simulink model "power_1phPWM"  (Simulink 6.0)
settings: Solver=VariableStepDiscrete  SolverMode=SingleTasking  StartTime=0.0  StopTime=0.1  MaxStep=Ts  RelTol=1e-3
InitFcn:
  | Ts=1/60/3240;
libraries: powerlib x28, powerlib_extras x3
settings Model: Creator=patrice  LastModifiedBy=batserve  ExtModeTrigMode=oneshot  ExtModeArmWhenConnect=off  ExtModeAutoUpdateStatusClock=off
settings DataIOCC: LimitDataPoints=off  SignalLoggingName=sigsOut
settings OptimizationCC: BlockReduction=off  BooleanDataType=off
settings DebuggingCC: CheckExecutionContextPreStartOutputMsg=on  CheckExecutionContextRuntimeOutputMsg=on  SolverPrmCheckMsg=none
settings HardwareCC: TargetUnknown=on
settings RTWCC: TemplateMakefile=grt_unix.tmf

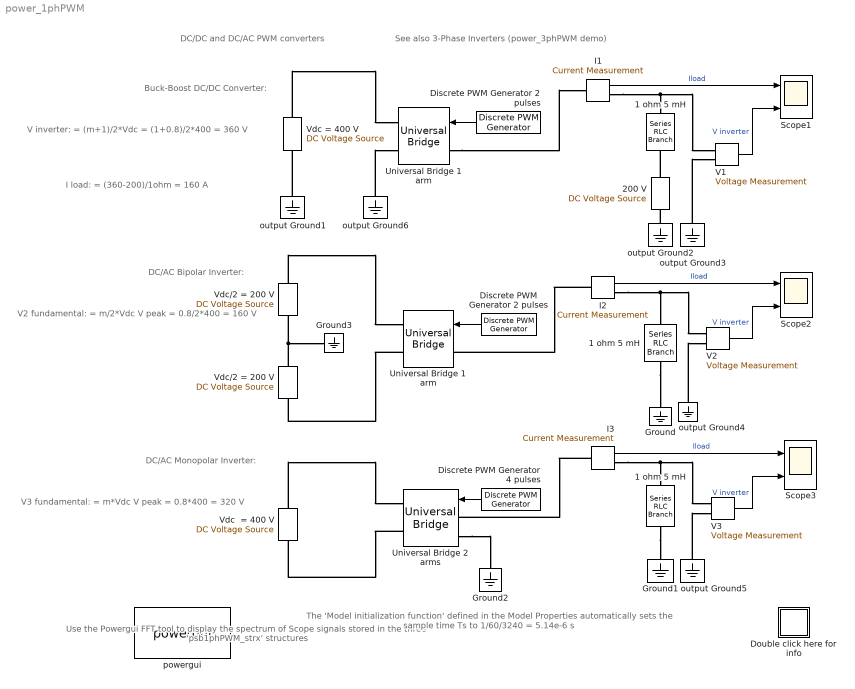
== system power_1phPWM ==
  note: V3 fundamental:
      |     = m*Vdc V peak
      |     = 0.8*400
      |     = 320 V
  note: DC/DC and DC/AC PWM converters
  note: V2 fundamental:
      |     = m/2*Vdc V peak
      |     = 0.8/2*400
      |     = 160 V
  note: V inverter:
      |     = (m+1)/2*Vdc
      |     = (1+0.8)/2*400
      |     = 360 V
  note: See also 3-Phase Inverters (power_3phPWM demo)
  note: Use the Powergui FFT tool to display the
      | spectrum of Scope  signals stored in the
      | three 'psb1phPWM_strx' structures
  note: Buck-Boost DC/DC Converter:
  note: DC/AC Bipolar Inverter:
  note: DC/AC Monopolar Inverter:
  note: I load:
      |     = (360-200)/1ohm
      |     = 160 A
  note: The 'Model  initialization function' defined in the
      | Model Properties automatically sets the sample time Ts
      | to 1/60/3240 = 5.14e-6 s
  1 ohm 5 mH : powerlib/Elements/Series RLC Branch  Orientation=down  PhysicalDomain=powersysdomain  SubClassName=unknown  LeftPortType=p1  RightPortType=p1  LConnTagsString=__new0  RConnTagsString=__new0  Resistance=1  Inductance=5e-03  Capacitance=inf  Measurements=None
  "1 ohm 5 mH " : powerlib/Elements/Series RLC Branch  Orientation=down  PhysicalDomain=powersysdomain  SubClassName=unknown  LeftPortType=p1  RightPortType=p1  LConnTagsString=__new0  RConnTagsString=__new0  Resistance=1  Inductance=5e-03  Capacitance=inf  Measurements=None
  "1 ohm 5 mH  " : powerlib/Elements/Series RLC Branch  Orientation=up  PhysicalDomain=powersysdomain  SubClassName=unknown  LeftPortType=p1  RightPortType=p1  LConnTagsString=__new0  RConnTagsString=__new0  Resistance=1  Inductance=5e-03  Capacitance=inf  Measurements=None
  200 V : powerlib/Electrical Sources/DC Voltage Source  Description=source block  Orientation=up  Amplitude=200  Measurements=None
      settings: AttributesFormatString=\n
  Discrete PWM Generator 2 pulses : powerlib_extras/Discrete  Control Blocks/Discrete PWM Generator  Orientation=left  GeneratorMode="1-arm  bridge (2 pulses)"  Fc=1080  Ts=Ts  Internal=on  mIndex=0.8  Freq=60  Phase=0
  "Discrete PWM Generator 2 pulses " : powerlib_extras/Discrete  Control Blocks/Discrete PWM Generator  Orientation=left  GeneratorMode="1-arm  bridge (2 pulses)"  Fc=1080  Ts=Ts  Internal=on  mIndex=0.8  Freq=0  Phase=0
  Discrete PWM Generator 4 pulses : powerlib_extras/Discrete  Control Blocks/Discrete PWM Generator  Orientation=left  GeneratorMode="2-arm  bridge (4 pulses)"  Fc=1080  Ts=Ts  Internal=on  mIndex=0.8  Freq=60  Phase=0
  Double click here for info : Subsystem
      mask Display: disp('?')
  Ground : powerlib/Elements/Ground  Orientation=down  PhysicalDomain=powersysdomain  SubClassName=unknown  LeftPortType=p1  RightPortType=p1  LConnTagsString=a
  Ground1 : powerlib/Elements/Ground  Orientation=down  PhysicalDomain=powersysdomain  SubClassName=unknown  LeftPortType=p1  RightPortType=p1  LConnTagsString=a
  Ground2 : powerlib/Elements/Ground  Orientation=down  PhysicalDomain=powersysdomain  SubClassName=unknown  LeftPortType=p1  RightPortType=p1  LConnTagsString=a
  Ground3 : powerlib/Elements/Ground  PhysicalDomain=powersysdomain  SubClassName=unknown  LeftPortType=p1  RightPortType=p1  LConnTagsString=a
  I1 : powerlib/Measurements/Current Measurement  Tag=PoWeRsYsTeMmEaSuReMeNt  PhasorSimulation=off  OutputType=Magnitude  PSBequivalent=0
  I2 : powerlib/Measurements/Current Measurement  Tag=PoWeRsYsTeMmEaSuReMeNt  PhasorSimulation=off  OutputType=Magnitude  PSBequivalent=0
  "I3 " : powerlib/Measurements/Current Measurement  Tag=PoWeRsYsTeMmEaSuReMeNt  PhasorSimulation=off  OutputType=Magnitude  PSBequivalent=0
  "Scope1 " : Scope  NumInputPorts=2
      settings: TimeRange=0.1  YMin=0~-50  YMax=175~400  SaveName=psb1phPWM1_str  MaxDataPoints=500000
  Scope2 : Scope  NumInputPorts=2
      settings: TimeRange=0.1  YMin=-100~-300  YMax=100~300  SaveName=psb1phPWM2_str  MaxDataPoints=500000
  Scope3 : Scope  NumInputPorts=2
      settings: TimeRange=0.1  YMin=-200~-500  YMax=200~500  SaveName=psb1phPWM3_str  MaxDataPoints=500000
  Universal Bridge 1 arm : powerlib/Power Electronics/Universal Bridge  Orientation=left  Arms=1  SnubberResistance=10000  SnubberCapacitance=inf  Device=IGBT / Diodes  Ron=1e-4  Lon=0  ForwardVoltages="[  1  1  ]"  ForwardVoltage=.8  GTOparameters=[ 10e-6 , 20e-6 ]  IGBTparameters=[ 1e-6 , 2e-6 ]  Measurements=None
  "Universal Bridge 1 arm " : powerlib/Power Electronics/Universal Bridge  Orientation=left  Arms=1  SnubberResistance=10000  SnubberCapacitance=inf  Device=IGBT / Diodes  Ron=1e-4  Lon=0  ForwardVoltages="[  1  1  ]"  ForwardVoltage=.8  GTOparameters=[ 10e-6 , 20e-6 ]  IGBTparameters=[ 1e-6 , 2e-6 ]  Measurements=None
  Universal Bridge 2 arms : powerlib/Power Electronics/Universal Bridge  Orientation=left  Arms=2  SnubberResistance=10000  SnubberCapacitance=inf  Device=IGBT / Diodes  Ron=1e-4  Lon=0  ForwardVoltages="[  1  1  ]"  ForwardVoltage=.8  GTOparameters=[ 10e-6 , 20e-6 ]  IGBTparameters=[ 1e-6 , 2e-6 ]  Measurements=None
  "V1 " : powerlib/Measurements/Voltage Measurement  Tag=PoWeRsYsTeMmEaSuReMeNt  PhasorSimulation=off  OutputType=Magnitude  PSBequivalent=0
  V2 : powerlib/Measurements/Voltage Measurement  Tag=PoWeRsYsTeMmEaSuReMeNt  PhasorSimulation=off  OutputType=Magnitude  PSBequivalent=0
  V3 : powerlib/Measurements/Voltage Measurement  Tag=PoWeRsYsTeMmEaSuReMeNt  PhasorSimulation=off  OutputType=Magnitude  PSBequivalent=0
  "Vdc  = 400 V  " : powerlib/Electrical Sources/DC Voltage Source  Description=source block  Orientation=up  Amplitude=400  Measurements=None
      settings: AttributesFormatString=\n
  Vdc = 400 V : powerlib/Electrical Sources/DC Voltage Source  Description=source block  Orientation=up  Amplitude=400  Measurements=None
      settings: AttributesFormatString=\n
  Vdc/2 = 200 V : powerlib/Electrical Sources/DC Voltage Source  Description=source block  Orientation=up  Amplitude=200  Measurements=None
      settings: AttributesFormatString=\n
  "Vdc/2 = 200 V " : powerlib/Electrical Sources/DC Voltage Source  Description=source block  Orientation=up  Amplitude=200  Measurements=None
      settings: AttributesFormatString=\n
  output Ground{1..6} (6 alike) : powerlib/Elements/Ground  Orientation=down  PhysicalDomain=powersysdomain  SubClassName=unknown  LeftPortType=p1  RightPortType=p1  LConnTagsString=a
  powergui : powerlib/powergui  Priority=2  Frange=[0:2:500]  Ylog=off  Xlog=off  save=off  variable=ZData  structure=psb1phPWM1_str  ZoomFFT=on  StartTime=0.1-2/60  cycles=2  DisplayStyle=off  fundamental=60  FreqAxis=off  MaxFrequency=5000  frequencyindice=1  frequencyindicesteady=1  RmsSteady=1  display=off  Ts=Ts  methode=off  frequency=60  echomessages=on
  wires:
  I1/1 -> "Scope1 "/1  "Iload"
  "Discrete PWM Generator 2 pulses "/1 -> Universal Bridge 1 arm/1
  I2/1 -> Scope2/1  "Iload"
  Discrete PWM Generator 2 pulses/1 -> "Universal Bridge 1 arm "/1
  V2/1 -> Scope2/2  "V inverter"
  Discrete PWM Generator 4 pulses/1 -> Universal Bridge 2 arms/1
  "I3 "/1 -> Scope3/1  "Iload"
  V3/1 -> Scope3/2  "V inverter"
  "V1 "/1 -> "Scope1 "/2  "V inverter"
  connections:
  Universal Bridge 1 arm/LConn1 -- I1/LConn1
  Vdc = 400 V/RConn1 -- Universal Bridge 1 arm/RConn1
  Vdc/2 = 200 V/RConn1 -- "Universal Bridge 1 arm "/RConn1
  I2/RConn1 -- 1 ohm 5 mH/LConn1 -- V2/LConn1
  "Vdc/2 = 200 V "/RConn1 -- Vdc/2 = 200 V/LConn1 -- Ground3/LConn1
  "I3 "/RConn1 -- "1 ohm 5 mH "/LConn1 -- V3/LConn1
  output Ground1/LConn1 -- Vdc = 400 V/LConn1
  200 V/RConn1 -- "1 ohm 5 mH  "/LConn1
  output Ground2/LConn1 -- 200 V/LConn1
  output Ground3/LConn1 -- "V1 "/LConn2
  1 ohm 5 mH/RConn1 -- Ground/LConn1
  output Ground4/LConn1 -- V2/LConn2
  "1 ohm 5 mH "/RConn1 -- Ground1/LConn1
  output Ground5/LConn1 -- V3/LConn2
  output Ground6/LConn1 -- Universal Bridge 1 arm/RConn2
  I1/RConn1 -- "1 ohm 5 mH  "/RConn1 -- "V1 "/LConn1
  "Universal Bridge 1 arm "/RConn2 -- "Vdc/2 = 200 V "/LConn1
  I2/LConn1 -- "Universal Bridge 1 arm "/LConn1
  Universal Bridge 2 arms/RConn2 -- "Vdc  = 400 V  "/LConn1
  "Vdc  = 400 V  "/RConn1 -- Universal Bridge 2 arms/RConn1
  Universal Bridge 2 arms/LConn2 -- Ground2/LConn1
  "I3 "/LConn1 -- Universal Bridge 2 arms/LConn1

== system power_1phPWM/Double click here for info ==
  note: G. Sybille and P. Giroux (Hydro-Quebec)
  note: Demonstration
  note: Circuit Description
  note: This demonstration illustrates use of the Universal Bridge and
      | Discrete PWM Pulse Generator blocks. It also demonstrates
      | harmonic analysis of PWM waveforms using the Powergui/FFT tool.
  note: The system consists of three independant circuits illustrating various PWM DC/DC and DC/AC inverters.
      | All converters are controlled in open loop with the Discrete PWM Generator block available in the Extras/Discrete Control Blocks library.
      | The three circuits use the same DC voltage (Vdc = 400V), carrier frequency (1080 Hz) and modulation index (m = 0.8) .
      | From top to bottom, the three circuits are:
      |
      | 1. DC/DC, two-quadrant converter (one-arm; two-switches)
      | 2. DC/AC,  bipolar converter  (one-arm; two-switches)
      | 3. DC/AC, monopolar  converter (two-arms; four-switches)
      |
      | In order to allow further signal processing, signals displayed on the three Scope blocks  (sampled at simulation sampling rate of 3240 samples/cycle)
      | are stored in three  variables named 'psb1phPWM1_str' , 'psb1phPWM2_str'  and  'psb1phPWM3_str'  (structures with time).
  note: Run the simulation and observe the following two waveforms on the Scope blocks:
      | current into the load (trace 1), voltage generated by the PWM inverter (trace 2).
      |
      | Once the  simulation is completed, open the Powergui and select 'FFT Analysis' to display the 0 - 5000 Hz frequency spectrum of signals saved
      | in the three 'psb1phPWMx_str' structures. The FFT will be performed on  a 2-cycle window starting at t = 0.1 - 2/60 (last 2 cycles of recording).
      | For each circuit selelect Input labeled 'V inverter' . Click on Display and observe the frequency spectrum of last 2 cycles.
      |
      | The fundamental component of  V inverter (DC component in case of circuit 1) is displayed above the spectrum window.
      | Compare the magnitude of the fundamental or DC component of the inverter voltage with the theoretical values given in the  circuit.
      | Compare also the harmonic contents in the inverter voltage for the two-switch and four-switch DC/AC inverters.
      |
      | For the two-switch inverter,  the first harmonics  occur around the carrier frequency (1080 Hz +- k*60 Hz, with a maximum of 103% at 1080 Hz ),
      | whereas for the four-switch inverter harmonics are lower and appear at double of carrier frequency (maximum of 40% at 2*1080+-60 Hz)
      |
      | As a result, the current is "cleaner" for the four-switch inverter.
      |
      | If you now perform a FFT on the signal Iload you will notice that the THD of load current is 7.3% for the two-switch inverter as compared to
      | only  2% for the four-switch inverter.
